simulink model "probSix"  (R2020b)
settings: Solver=VariableStepDiscrete  StartTime=0.0  StopTime=10.0  MaxStep=0.1  RelTol=1e-3
libraries: simulink x1
settings Model: Creator='Z'ome  LastModifiedBy='Z'ome

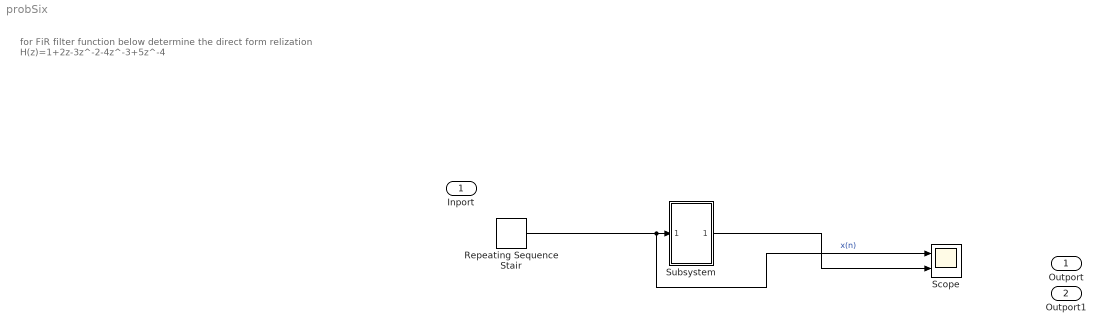
== system probSix ==
  note: for FiR filter function below determine the direct form relization
      | H(z)=1+2z-3z^-2-4z^-3+5z^-4
  Inport : Inport
  Repeating Sequence Stair : simulink/Sources/Repeating Sequence Stair  OutValues=[1 0 0 0 0 0 0 0 0].'  tsamp=-1  OutMin=[]  OutMax=[]  OutDataTypeStr=double  OutputDataTypeScalingMode=double  OutDataType=fixdt(0,8)  ConRadixGroup=Best Precision: Vector-wise  OutScaling=2^-12
  Scope : Scope  NumInputPorts=2
  Subsystem : Subsystem  TreatAsAtomicUnit=on
  Outport : Outport
  Outport1 : Outport  Port=2
  wires:
  Repeating Sequence Stair/1 -> Scope/1, Subsystem/1(x(n))  "x(n)"
  Subsystem/1(y(n)) -> Scope/2

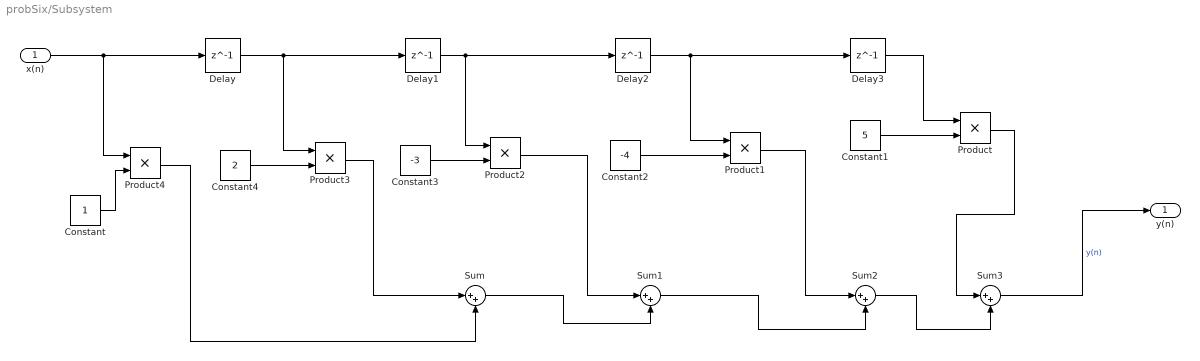
== system probSix/Subsystem ==
  x(n) : Inport
  Constant : Constant
  Constant1 : Constant  Value=5
  Constant2 : Constant  Value=-4
  Constant3 : Constant  Value=-3
  Constant4 : Constant  Value=2
  Delay{,1..3} (4 alike) : Delay  DelayLength=1
  Product{,1..4} (5 alike) : Product
  Sum{,1..3} (4 alike) : Sum  Inputs=|++
  y(n) : Outport
  wires:
  Constant4/1 -> Product3/2
  Constant1/1 -> Product/2
  Sum/1 -> Sum1/2
  Delay/1 -> Delay1/1, Product3/1
  Constant/1 -> Product4/2
  Product4/1 -> Sum/2
  Constant3/1 -> Product2/2
  Sum1/1 -> Sum2/2
  Delay1/1 -> Delay2/1, Product2/1
  Product2/1 -> Sum1/1
  Constant2/1 -> Product1/2
  Sum2/1 -> Sum3/2
  Product/1 -> Sum3/1
  x(n)/1 -> Delay/1, Product4/1
  Product1/1 -> Sum2/1
  Product3/1 -> Sum/1
  Delay3/1 -> Product/1
  Delay2/1 -> Delay3/1, Product1/1
  Sum3/1 -> y(n)/1  "y(n)"
